simulink model "srmob_lab_model"  (R2018a)
settings: Solver=ode45  StartTime=0.0  StopTime=t_end  FixedStep=t_pp  MaxStep=t_pp  RelTol=1e-3
values from neighbouring files (symbols this model uses):
  inv_J = inv(J)    [srmob_lab_init.m]
  inv_N = inv(N)    [srmob_lab_init.m]
  inv_R_m = inv(R_m)    [srmob_lab_init.m]
  k_c = k_i+50    (= 115.65867657)    [srmob_lab_init.m]
  k_i = (T*omega_0^2) / (K*k_p)    (= 65.6586765699)    [srmob_lab_init.m]
  K_m = [k_m 0; 0 k_m]    [srmob_lab_init.m]
  k_p = (2*T*zeta_0*omega_0 - 1) / K    (= 2.52443181818)    [srmob_lab_init.m]
  q_initial_conditions = [0; 0; -0.5]    [srmob_lab_init.m]
  T_F = 1/k_i    (= 0.0152302795646)    [srmob_lab_init.m]
  u_initial_conditions = [0; 0]    [srmob_lab_init.m]
  u_max = [u_limit; u_limit]    [srmob_lab_init.m]
  u_min = [-u_limit; -u_limit]    [srmob_lab_init.m]
settings Model: Creator=szymon  LastModifiedBy=tomas

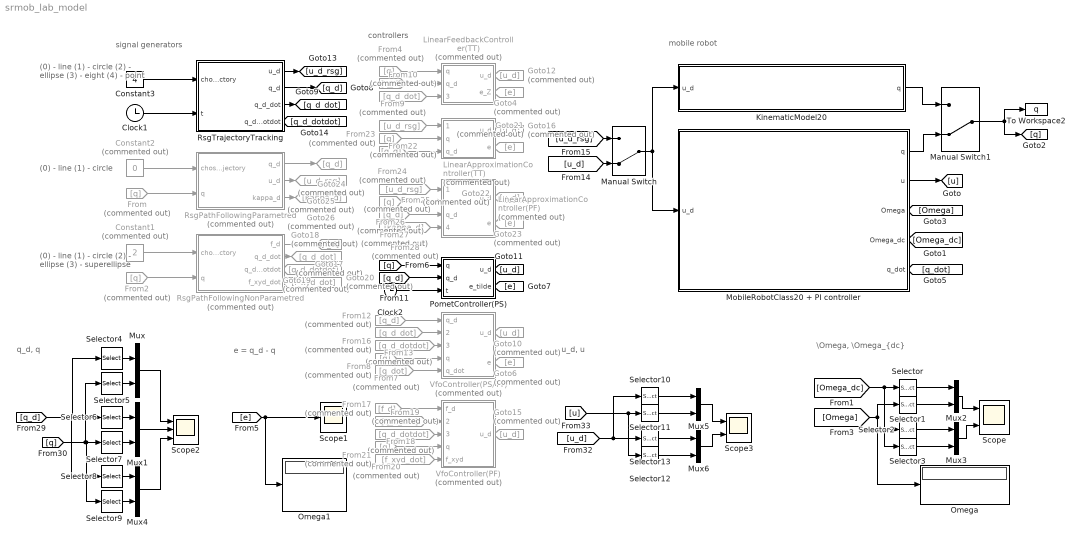
== system srmob_lab_model ==
  note: e = q_d - q
  note: signal generators
  note: controllers
  note: \Omega, \Omega_{dc}
  note: (0) - line
      | (1) - circle
      | (2) - ellipse
      | (3) - eight
      | (4) - point
  note: mobile robot
  note: (0) - line
      | (1) - circle
  note: (0) - line
      | (1) - circle
      | (2) - ellipse
      | (3) - superellipse
  note: q_d, q
  note: u_d, u
  Clock1 : Clock
  Clock2 : Clock
  Constant1 : Constant  Commented=on  Value=2
  Constant2 : Constant  Commented=on  Value=0
  Constant3 : Constant  Value=4
  From{,2,4,7,20,23,26} (7 alike) : From  Commented=on  GotoTag=q
  From10 : From  Commented=on  GotoTag=q_d_dot
  From{9,12,24,27} (4 alike) : From  Commented=on  GotoTag=q_d
  From13 : From  Commented=on  GotoTag=q_d_dot
  From16 : From  Commented=on  GotoTag=q_d_dotdot
  From17 : From  Commented=on  GotoTag=f_d
  From18 : From  Commented=on  GotoTag=q_d_dot
  From19 : From  Commented=on  GotoTag=q_d_dotdot
  From21 : From  Commented=on  GotoTag=f_xyd_dot
  From22 : From  Commented=on  GotoTag=u_d_rsg
  From25 : From  Commented=on  GotoTag=u_d_rsg
  From28 : From  Commented=on  GotoTag=kappa_d
  From8 : From  Commented=on  GotoTag=q_dot
  Goto{10,12,15..16,22} (5 alike) : Goto  Commented=on  GotoTag=u_d
  Goto17 : Goto  Commented=on  GotoTag=f_d
  Goto18 : Goto  Commented=on  GotoTag=q_d_dot
  Goto19 : Goto  Commented=on  GotoTag=q_d_dotdot
  Goto20 : Goto  Commented=on  GotoTag=f_xyd_dot
  Goto{4,6,21,23} (4 alike) : Goto  Commented=on  GotoTag=e
  Goto24 : Goto  Commented=on  GotoTag=q_d
  Goto25 : Goto  Commented=on  GotoTag=u_d_rsg
  Goto26 : Goto  Commented=on  GotoTag=kappa_d
  KinematicModel20 : Subsystem
  LinearApproximationController(PF) : Subsystem  Commented=on
  LinearApproximationController(TT) : Subsystem  Commented=on
  LinearFeedbackController(TT) : Subsystem  Commented=on
  Manual Switch : ManualSwitch  CurrentSetting=0
  Manual Switch1 : ManualSwitch  CurrentSetting=0
  MobileRobotClass20 + PI controller : Subsystem
  Mux{,1..6} (7 alike) : Mux  Inputs=2
  Omega : Display
  Omega1 : Display
  PometController(PS) : Subsystem
  RsgPathFollowingNonParametred : Subsystem  Commented=on
  RsgPathFollowingParametred : Subsystem  Commented=on
  RsgTrajectoryTracking : Subsystem
  Scope : Scope  NumInputPorts=2
  Scope1 : Scope
  Scope2 : Scope  NumInputPorts=3
  Scope3 : Scope  NumInputPorts=2
  Selector{,1,10..11} (4 alike) : Selector  InputPortWidth=2  IndexOptions=Index vector (dialog)  Indices=1  OutputSizes=1
  Selector{2..3,12..13} (4 alike) : Selector  InputPortWidth=2  IndexOptions=Index vector (dialog)  Indices=2  OutputSizes=1
  Selector4 : Selector  InputPortWidth=3  IndexOptions=Index vector (dialog)  Indices=1  OutputSizes=1
  Selector5 : Selector  InputPortWidth=3  IndexOptions=Index vector (dialog)  Indices=1  OutputSizes=1
  Selector6 : Selector  InputPortWidth=3  IndexOptions=Index vector (dialog)  Indices=2  OutputSizes=1
  Selector7 : Selector  InputPortWidth=3  IndexOptions=Index vector (dialog)  Indices=2  OutputSizes=1
  Selector8 : Selector  InputPortWidth=3  IndexOptions=Index vector (dialog)  Indices=3  OutputSizes=1
  Selector9 : Selector  InputPortWidth=3  IndexOptions=Index vector (dialog)  Indices=3  OutputSizes=1
  To Workspace2 : ToWorkspace  VariableName=q  SampleTime=-1
  VfoController(PF) : Subsystem  Commented=on
  VfoController(PS/TT) : Subsystem  Commented=on
  wires:
  Selector/1 -> Mux2/1
  Selector1/1 -> Mux2/2
  Selector2/1 -> Mux3/1
  Selector3/1 -> Mux3/2
  Mux2/1 -> Scope/1
  Clock1/1 -> RsgTrajectoryTracking/2(t)
  From/1 -> RsgPathFollowingParametred/2(q)
  MobileRobotClass20 + PI controller/1(q) -> Manual Switch1/2
  MobileRobotClass20 + PI controller/2(u) -> [u]
  MobileRobotClass20 + PI controller/4(Omega_dc) -> [Omega_dc]
  From2/1 -> RsgPathFollowingNonParametred/2(q)
  MobileRobotClass20 + PI controller/3(Omega) -> [Omega]
  Constant1/1 -> RsgPathFollowingNonParametred/1(chosen_trajectory)
  Constant2/1 -> RsgPathFollowingParametred/1(chosen_trajectory)
  Constant3/1 -> RsgTrajectoryTracking/1(chosen_trajectory)
  Manual Switch1/1 -> To Workspace2/1, [q]
  From4/1 -> LinearFeedbackController(TT)/1(q)
  Manual Switch/1 -> KinematicModel20/1(u_d), MobileRobotClass20 + PI controller/1(u_d)
  LinearFeedbackController(TT)/2(e_Z) -> Goto4/1
  [e] -> Scope1/1, Omega1/1
  Mux3/1 -> Scope/2
  [Omega_dc] -> Selector3/1, Selector/1
  [Omega] -> Omega/1, Selector2/1, Selector1/1
  Clock2/1 -> PometController(PS)/3(t)
  [q] -> PometController(PS)/1(q)
  From7/1 -> VfoController(PS/TT)/4(q)
  PometController(PS)/1(u_d) -> [u_d]
  MobileRobotClass20 + PI controller/5(q_dot) -> [q_dot]
  From8/1 -> VfoController(PS/TT)/5(q_dot)
  VfoController(PS/TT)/2(e) -> Goto6/1
  PometController(PS)/2(e_tilde) -> [e]
  RsgTrajectoryTracking/2(q_d) -> [q_d]
  From9/1 -> LinearFeedbackController(TT)/2(q_d)
  RsgTrajectoryTracking/3(q_d_dot) -> [q_d_dot]
  From10/1 -> LinearFeedbackController(TT)/3(q_d_dot)
  [q_d] -> PometController(PS)/2(q_d)
  From12/1 -> VfoController(PS/TT)/1(q_d)
  From13/1 -> VfoController(PS/TT)/2(q_d_dot)
  VfoController(PS/TT)/1(u_d) -> Goto10/1
  LinearFeedbackController(TT)/1(u_d) -> Goto12/1
  [u_d] -> Manual Switch/2
  RsgTrajectoryTracking/1(u_d) -> [u_d_rsg]
  [u_d_rsg] -> Manual Switch/1
  KinematicModel20/1(q) -> Manual Switch1/1
  RsgTrajectoryTracking/4(q_d_dotdot) -> [q_d_dotdot]
  From16/1 -> VfoController(PS/TT)/3(q_d_dotdot)
  RsgPathFollowingNonParametred/2(q_d_dot) -> Goto18/1
  RsgPathFollowingNonParametred/3(q_d_dotdot) -> Goto19/1
  RsgPathFollowingNonParametred/1(f_d) -> Goto17/1
  From18/1 -> VfoController(PF)/2(q_d_dot)
  From19/1 -> VfoController(PF)/3(q_d_dotdot)
  From17/1 -> VfoController(PF)/1(f_d)
  From20/1 -> VfoController(PF)/4(q)
  RsgPathFollowingNonParametred/4(f_xyd_dot) -> Goto20/1
  From21/1 -> VfoController(PF)/5(f_xyd)
  VfoController(PF)/1(u_d) -> Goto15/1
  From23/1 -> LinearApproximationController(TT)/2(q)
  LinearApproximationController(TT)/1(u_d) -> Goto16/1
  LinearApproximationController(TT)/2(e) -> Goto21/1
  From24/1 -> LinearApproximationController(TT)/3(q_d)
  From22/1 -> LinearApproximationController(TT)/1(u_d_rsg)
  LinearApproximationController(PF)/1(u_d) -> Goto22/1
  LinearApproximationController(PF)/2(e) -> Goto23/1
  RsgPathFollowingParametred/1(q_d) -> Goto24/1
  RsgPathFollowingParametred/2(u_d) -> Goto25/1
  RsgPathFollowingParametred/3(kappa_d) -> Goto26/1
  From25/1 -> LinearApproximationController(PF)/1(u_d_rsg)
  From26/1 -> LinearApproximationController(PF)/2(q)
  From27/1 -> LinearApproximationController(PF)/3(q_d)
  From28/1 -> LinearApproximationController(PF)/4(kappa_d)
  [q_d] -> Selector8/1, Selector4/1, Selector6/1
  Selector4/1 -> Mux/1
  Selector5/1 -> Mux/2
  Mux/1 -> Scope2/1
  Selector7/1 -> Mux1/2
  Mux1/1 -> Scope2/2
  Selector6/1 -> Mux1/1
  Selector9/1 -> Mux4/2
  Mux4/1 -> Scope2/3
  Selector8/1 -> Mux4/1
  [q] -> Selector5/1, Selector9/1, Selector7/1
  Selector13/1 -> Mux6/1
  Selector10/1 -> Mux5/1
  Mux6/1 -> Scope3/2
  Selector11/1 -> Mux5/2
  Mux5/1 -> Scope3/1
  Selector12/1 -> Mux6/2
  [u_d] -> Selector10/1, Selector13/1
  [u] -> Selector12/1, Selector11/1

== system srmob_lab_model/KinematicModel20 ==
  u_d : Inport
  Demux : Demux  Outputs=3
  Integrator : Integrator  InitialCondition=q_initial_conditions
  KinematicModel : MATLABFcn  MATLABFcn=KinematicModel
  Mux : Mux  Inputs=2
  Mux1 : Mux  Inputs=3
  q : Outport
  wires:
  KinematicModel/1 -> Integrator/1  "q'"
  Mux/1 -> KinematicModel/1
  u_d/1 -> Mux/2
  Integrator/1 -> Demux/1  "q"
  Demux/1 -> Mux/1, Mux1/1  "theta"
  Demux/3 -> Mux1/3  "y"
  Demux/2 -> Mux1/2  "x"
  Mux1/1 -> q/1

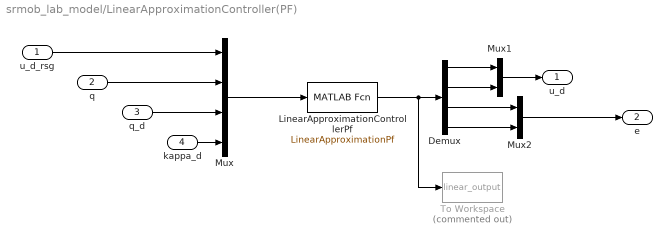
== system srmob_lab_model/LinearApproximationController(PF) ==
  u_d_rsg : Inport
  q : Inport  Port=2
  q_d : Inport  Port=3
  kappa_d : Inport  Port=4
  Demux : Demux
  LinearApproximationControllerPf : MATLABFcn  MATLABFcn=LinearApproximationPf
  Mux : Mux
  Mux1 : Mux  Inputs=2
  Mux2 : Mux  Inputs=2
  To Workspace : ToWorkspace  Commented=on  VariableName=linear_output  SampleTime=-1
  u_d : Outport
  e : Outport  Port=2
  wires:
  Mux/1 -> LinearApproximationControllerPf/1
  q_d/1 -> Mux/3
  LinearApproximationControllerPf/1 -> Demux/1, To Workspace/1
  Demux/1 -> Mux1/1
  Demux/2 -> Mux1/2
  Mux2/1 -> e/1
  Mux1/1 -> u_d/1
  u_d_rsg/1 -> Mux/1
  q/1 -> Mux/2
  kappa_d/1 -> Mux/4
  Demux/4 -> Mux2/2
  Demux/3 -> Mux2/1

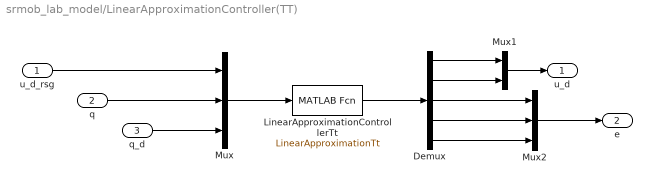
== system srmob_lab_model/LinearApproximationController(TT) ==
  u_d_rsg : Inport
  q : Inport  Port=2
  q_d : Inport  Port=3
  Demux : Demux  Outputs=5
  LinearApproximationControllerTt : MATLABFcn  MATLABFcn=LinearApproximationTt
  Mux : Mux  Inputs=3
  Mux1 : Mux  Inputs=2
  Mux2 : Mux  Inputs=3
  u_d : Outport
  e : Outport  Port=2
  wires:
  Mux/1 -> LinearApproximationControllerTt/1
  q_d/1 -> Mux/3
  LinearApproximationControllerTt/1 -> Demux/1
  Demux/1 -> Mux1/1
  Demux/2 -> Mux1/2
  Demux/3 -> Mux2/1
  Demux/4 -> Mux2/2
  Mux2/1 -> e/1
  Mux1/1 -> u_d/1
  u_d_rsg/1 -> Mux/1
  q/1 -> Mux/2
  Demux/5 -> Mux2/3

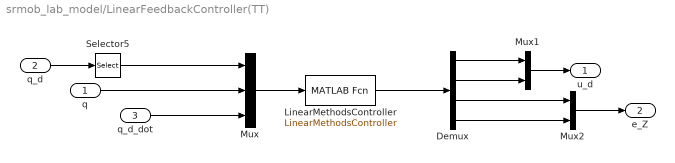
== system srmob_lab_model/LinearFeedbackController(TT) ==
  q : Inport
  q_d : Inport  Port=2
  q_d_dot : Inport  Port=3
  Demux : Demux
  LinearMethodsController : MATLABFcn  MATLABFcn=LinearMethodsController
  Mux : Mux  Inputs=3
  Mux1 : Mux  Inputs=2
  Mux2 : Mux  Inputs=2
  Selector5 : Selector  InputPortWidth=3  IndexOptions=Index vector (dialog)  Indices=[2 3]  OutputSizes=1
  u_d : Outport
  e_Z : Outport  Port=2
  wires:
  Mux/1 -> LinearMethodsController/1
  q/1 -> Mux/2
  q_d/1 -> Selector5/1
  LinearMethodsController/1 -> Demux/1
  q_d_dot/1 -> Mux/3
  Demux/1 -> Mux1/1
  Demux/2 -> Mux1/2
  Demux/3 -> Mux2/1
  Demux/4 -> Mux2/2
  Mux2/1 -> e_Z/1
  Mux1/1 -> u_d/1
  Selector5/1 -> Mux/1

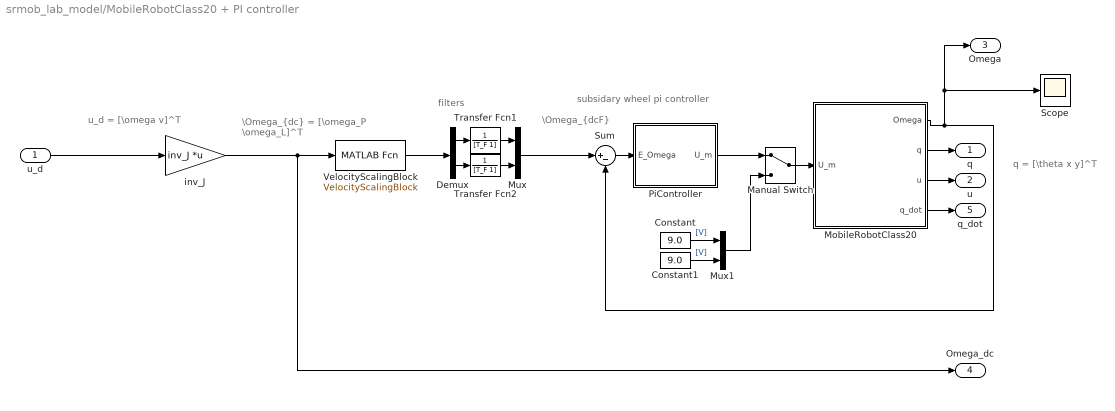
== system srmob_lab_model/MobileRobotClass20 + PI controller ==
  note: q = [\theta x y]^T
  note: u_d = [\omega v]^T
  note: \Omega_{dc} = [\omega_P \omega_L]^T
  note: \Omega_{dcF}
  note: subsidary wheel pi controller
  note: filters
  u_d : Inport
  Constant : Constant  Value=9.0
  Constant1 : Constant  Value=9.0
  Demux : Demux  Outputs=2
  Manual Switch : ManualSwitch
  MobileRobotClass20 : Subsystem
  Mux : Mux  Inputs=2
  Mux1 : Mux  Inputs=2
  PiController : Subsystem
  Scope : Scope
  Sum : Sum  Inputs=|+-
  Transfer Fcn1 : TransferFcn  Numerator=1  Denominator=[T_F 1]
  Transfer Fcn2 : TransferFcn  Numerator=1  Denominator=[T_F 1]
  VelocityScalingBlock : MATLABFcn  MATLABFcn=VelocityScalingBlock
  inv_J : Gain  Gain=inv_J  Multiplication=Matrix(K*u)
  q : Outport
  u : Outport  Port=2
  Omega : Outport  Port=3
  Omega_dc : Outport  Port=4
  q_dot : Outport  Port=5
  wires:
  Demux/1 -> Transfer Fcn1/1
  Transfer Fcn1/1 -> Mux/1
  Transfer Fcn2/1 -> Mux/2
  u_d/1 -> inv_J/1
  Constant/1 -> Mux1/1  "[V]"
  MobileRobotClass20/2(q) -> q/1
  Demux/2 -> Transfer Fcn2/1
  Manual Switch/1 -> MobileRobotClass20/1(U_m)
  Sum/1 -> PiController/1(E_Omega)
  MobileRobotClass20/3(u) -> u/1
  MobileRobotClass20/1(Omega) -> Omega/1, Scope/1, Sum/2
  Mux1/1 -> Manual Switch/2
  PiController/1(U_m) -> Manual Switch/1
  Mux/1 -> Sum/1
  VelocityScalingBlock/1 -> Demux/1
  Constant1/1 -> Mux1/2  "[V]"
  inv_J/1 -> Omega_dc/1, VelocityScalingBlock/1
  MobileRobotClass20/4(q_dot) -> q_dot/1

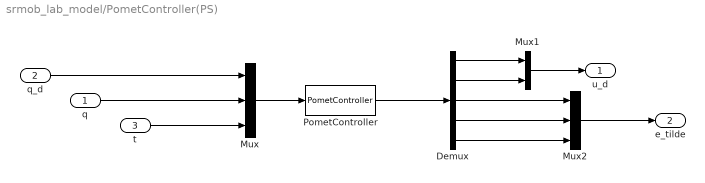
== system srmob_lab_model/PometController(PS) ==
  q : Inport
  q_d : Inport  Port=2
  t : Inport  Port=3
  Demux : Demux  Outputs=5
  Mux : Mux  Inputs=3
  Mux1 : Mux  Inputs=2
  Mux2 : Mux  Inputs=3
  PometController : MATLABFcn  MATLABFcn=PometController
  u_d : Outport
  e_tilde : Outport  Port=2
  wires:
  Mux/1 -> PometController/1
  q/1 -> Mux/2
  q_d/1 -> Mux/1
  PometController/1 -> Demux/1
  t/1 -> Mux/3
  Demux/1 -> Mux1/1
  Demux/2 -> Mux1/2
  Demux/3 -> Mux2/1
  Demux/4 -> Mux2/2
  Mux2/1 -> e_tilde/1
  Mux1/1 -> u_d/1
  Demux/5 -> Mux2/3

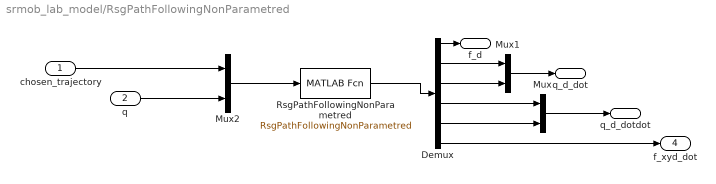
== system srmob_lab_model/RsgPathFollowingNonParametred ==
  chosen_trajectory : Inport
  q : Inport  Port=2
  Demux : Demux  Outputs=6
  Mux : Mux  Inputs=2
  Mux1 : Mux  Inputs=2
  Mux2 : Mux  Inputs=2
  RsgPathFollowingNonParametred : MATLABFcn  MATLABFcn=RsgPathFollowingNonParametred
  f_d : Outport
  q_d_dot : Outport  Port=2
  q_d_dotdot : Outport  Port=3
  f_xyd_dot : Outport  Port=4
  wires:
  RsgPathFollowingNonParametred/1 -> Demux/1
  q/1 -> Mux2/2
  chosen_trajectory/1 -> Mux2/1
  Mux2/1 -> RsgPathFollowingNonParametred/1
  Mux/1 -> q_d_dotdot/1
  Demux/2 -> Mux1/1
  Demux/3 -> Mux1/2
  Demux/4 -> Mux/1
  Demux/5 -> Mux/2
  Demux/1 -> f_d/1
  Mux1/1 -> q_d_dot/1
  Demux/6 -> f_xyd_dot/1

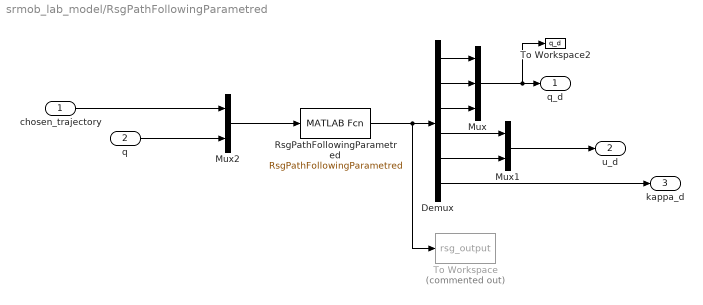
== system srmob_lab_model/RsgPathFollowingParametred ==
  chosen_trajectory : Inport
  q : Inport  Port=2
  Demux : Demux  Outputs=6
  Mux : Mux  Inputs=3
  Mux1 : Mux  Inputs=2
  Mux2 : Mux  Inputs=2
  RsgPathFollowingParametred : MATLABFcn  MATLABFcn=RsgPathFollowingParametred
  To Workspace : ToWorkspace  Commented=on  VariableName=rsg_output  SampleTime=-1
  To Workspace2 : ToWorkspace  VariableName=q_d  SampleTime=-1
  q_d : Outport
  u_d : Outport  Port=2
  kappa_d : Outport  Port=3
  wires:
  RsgPathFollowingParametred/1 -> Demux/1, To Workspace/1
  Demux/1 -> Mux/1
  Demux/2 -> Mux/2
  Demux/3 -> Mux/3
  Demux/5 -> Mux1/2
  Demux/4 -> Mux1/1
  Mux1/1 -> u_d/1
  q/1 -> Mux2/2
  chosen_trajectory/1 -> Mux2/1
  Mux2/1 -> RsgPathFollowingParametred/1
  Demux/6 -> kappa_d/1
  Mux/1 -> To Workspace2/1, q_d/1

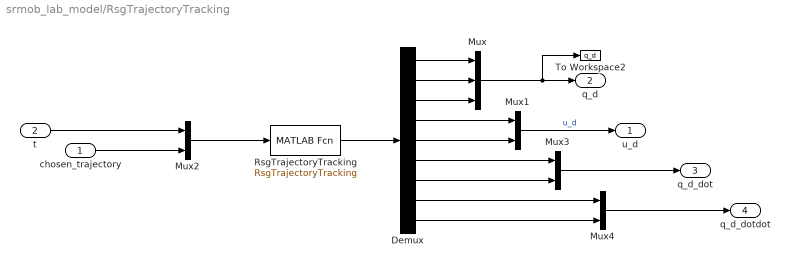
== system srmob_lab_model/RsgTrajectoryTracking ==
  chosen_trajectory : Inport
  t : Inport  Port=2
  Demux : Demux  Outputs=9
  Mux : Mux  Inputs=3
  Mux{1..4} (4 alike) : Mux  Inputs=2
  RsgTrajectoryTracking : MATLABFcn  MATLABFcn=RsgTrajectoryTracking
  To Workspace2 : ToWorkspace  VariableName=q_d  SampleTime=-1
  u_d : Outport
  q_d : Outport  Port=2
  q_d_dot : Outport  Port=3
  q_d_dotdot : Outport  Port=4
  wires:
  t/1 -> Mux2/1
  RsgTrajectoryTracking/1 -> Demux/1
  Demux/1 -> Mux/1
  Demux/2 -> Mux/2
  Demux/3 -> Mux/3
  Mux/1 -> To Workspace2/1, q_d/1
  Demux/5 -> Mux1/2
  Demux/4 -> Mux1/1
  Mux1/1 -> u_d/1  "u_d"
  Mux2/1 -> RsgTrajectoryTracking/1
  chosen_trajectory/1 -> Mux2/2
  Demux/7 -> Mux3/2
  Demux/6 -> Mux3/1
  Mux3/1 -> q_d_dot/1
  Demux/9 -> Mux4/2
  Demux/8 -> Mux4/1
  Mux4/1 -> q_d_dotdot/1

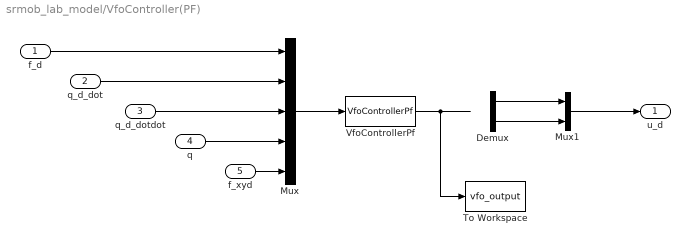
== system srmob_lab_model/VfoController(PF) ==
  f_d : Inport
  q_d_dot : Inport  Port=2
  q_d_dotdot : Inport  Port=3
  q : Inport  Port=4
  f_xyd : Inport  Port=5
  Demux : Demux  Outputs=2
  Mux : Mux  Inputs=5
  Mux1 : Mux  Inputs=2
  To Workspace : ToWorkspace  VariableName=vfo_output  SampleTime=-1
  VfoControllerPf : MATLABFcn  MATLABFcn=VfoControllerPf
  u_d : Outport
  wires:
  Mux/1 -> VfoControllerPf/1
  q_d_dot/1 -> Mux/2
  f_d/1 -> Mux/1
  VfoControllerPf/1 -> To Workspace/1
  q_d_dotdot/1 -> Mux/3
  Demux/1 -> Mux1/1
  Demux/2 -> Mux1/2
  Mux1/1 -> u_d/1
  q/1 -> Mux/4
  f_xyd/1 -> Mux/5

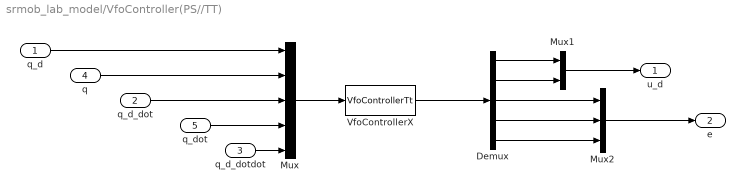
== system srmob_lab_model/VfoController(PS//TT) ==
  q_d : Inport
  q_d_dot : Inport  Port=2
  q_d_dotdot : Inport  Port=3
  q : Inport  Port=4
  q_dot : Inport  Port=5
  Demux : Demux  Outputs=5
  Mux : Mux  Inputs=5
  Mux1 : Mux  Inputs=2
  Mux2 : Mux  Inputs=3
  VfoControllerX : MATLABFcn  MATLABFcn=VfoControllerTt
  u_d : Outport
  e : Outport  Port=2
  wires:
  Mux/1 -> VfoControllerX/1
  q/1 -> Mux/2
  q_d/1 -> Mux/1
  VfoControllerX/1 -> Demux/1
  q_d_dot/1 -> Mux/3
  Demux/1 -> Mux1/1
  Demux/2 -> Mux1/2
  q_dot/1 -> Mux/4
  Mux1/1 -> u_d/1
  Demux/4 -> Mux2/2
  Demux/3 -> Mux2/1
  Mux2/1 -> e/1
  q_d_dotdot/1 -> Mux/5
  Demux/5 -> Mux2/3

== system srmob_lab_model/MobileRobotClass20 + PI controller/MobileRobotClass20 ==
  U_m : Inport
  DynamicModel : Subsystem
  KinematicModel : Subsystem
  Omega : Outport
  q : Outport  Port=2
  u : Outport  Port=3
  q_dot : Outport  Port=4
  wires:
  KinematicModel/1(q) -> q/1
  DynamicModel/1(Omega) -> Omega/1
  U_m/1 -> DynamicModel/1(U_m)
  DynamicModel/2(u_d) -> u/1, KinematicModel/1(u_d)
  KinematicModel/2(q_dot) -> q_dot/1

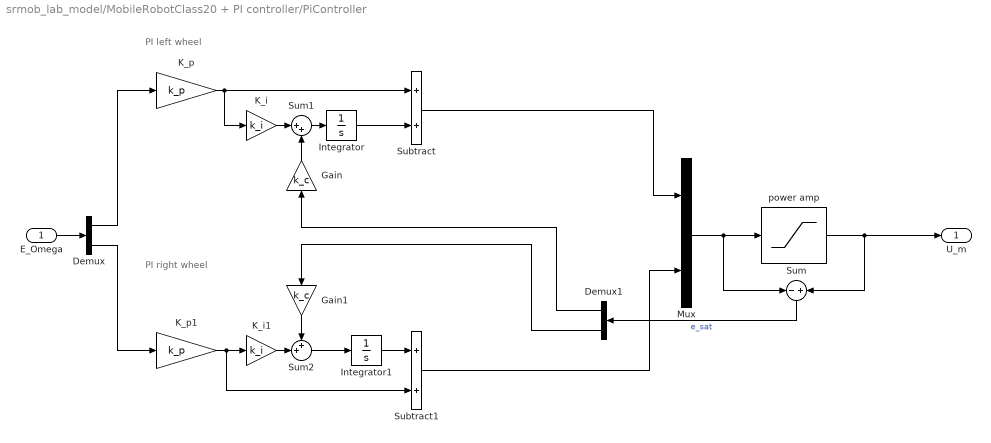
== system srmob_lab_model/MobileRobotClass20 + PI controller/PiController ==
  note: PI left wheel
  note: PI right wheel
  E_Omega : Inport
  Demux : Demux  Outputs=2
  Demux1 : Demux  Outputs=2
  Gain : Gain  Gain=k_c
  Gain1 : Gain  Gain=k_c
  Integrator : Integrator  InitialCondition=[0]
  Integrator1 : Integrator  InitialCondition=[0]
  K_i : Gain  Gain=k_i
  K_i1 : Gain  Gain=k_i
  K_p : Gain  Gain=k_p
  K_p1 : Gain  Gain=k_p
  Mux : Mux  Inputs=2
  Subtract : Sum
  Subtract1 : Sum
  Sum : Sum  Inputs=-+
  Sum1 : Sum  Inputs=|++
  Sum2 : Sum  Inputs=++|
  power amp : Saturate  UpperLimit=u_max  LowerLimit=u_min
  U_m : Outport
  wires:
  Demux/1 -> K_p/1
  Subtract/1 -> Mux/1
  K_i/1 -> Sum1/1
  K_p/1 -> K_i/1, Subtract/1
  Integrator/1 -> Subtract/2
  Demux/2 -> K_p1/1
  Subtract1/1 -> Mux/2
  K_p1/1 -> Subtract1/2, K_i1/1
  Integrator1/1 -> Subtract1/1
  Mux/1 -> Sum/1, power amp/1
  E_Omega/1 -> Demux/1
  power amp/1 -> Sum/2, U_m/1
  Sum/1 -> Demux1/1  "e_sat"
  Sum1/1 -> Integrator/1
  Demux1/1 -> Gain/1
  Sum2/1 -> Integrator1/1
  Gain/1 -> Sum1/2
  Demux1/2 -> Gain1/1
  K_i1/1 -> Sum2/2
  Gain1/1 -> Sum2/1

== system srmob_lab_model/MobileRobotClass20 + PI controller/MobileRobotClass20/DynamicModel ==
  U_m : Inport
  DynamicModel : MATLABFcn  MATLABFcn=DynamicModel
  Integrator : Integrator  InitialCondition=u_initial_conditions
  Mux : Mux  Inputs=2
  VoltageTorqueCalc : Subsystem
  inv_J : Gain  Gain=inv_J  Multiplication=Matrix(K*u) (u vector)
  power amp : Saturate  UpperLimit=u_max  LowerLimit=u_min
  Omega : Outport
  u_d : Outport  Port=2
  wires:
  Mux/1 -> DynamicModel/1
  DynamicModel/1 -> Integrator/1  "u'_d"
  Integrator/1 -> Mux/1, VoltageTorqueCalc/1(u), inv_J/1, u_d/1  "u"
  U_m/1 -> power amp/1
  inv_J/1 -> Omega/1
  VoltageTorqueCalc/1(T_m) -> Mux/2
  power amp/1 -> VoltageTorqueCalc/2(U_m)

== system srmob_lab_model/MobileRobotClass20 + PI controller/MobileRobotClass20/KinematicModel ==
  u_d : Inport
  Demux : Demux  Outputs=3
  Integrator : Integrator  InitialCondition=q_initial_conditions
  KinematicModel : MATLABFcn  MATLABFcn=KinematicModel
  Mux : Mux  Inputs=2
  Mux1 : Mux  Inputs=3
  q : Outport
  q_dot : Outport  Port=2
  wires:
  KinematicModel/1 -> q_dot/1, Integrator/1  "q'"
  Mux/1 -> KinematicModel/1
  u_d/1 -> Mux/2
  Integrator/1 -> Demux/1  "q"
  Demux/1 -> Mux/1, Mux1/1  "theta"
  Demux/3 -> Mux1/3  "y"
  Demux/2 -> Mux1/2  "x"
  Mux1/1 -> q/1

== system srmob_lab_model/MobileRobotClass20 + PI controller/MobileRobotClass20/DynamicModel/VoltageTorqueCalc ==
  u : Inport
  U_m : Inport  Port=2
  Gain : Gain  Gain=inv_N  Multiplication=Matrix(K*u) (u vector)
  Gain1 : Gain  Gain=K_m  Multiplication=Matrix(K*u) (u vector)
  K_m : Gain  Gain=K_m  Multiplication=Matrix(K*u) (u vector)
  Sum : Sum  Inputs=|+-
  inv_J : Gain  Gain=inv_J  Multiplication=Matrix(K*u) (u vector)
  inv_R : Gain  Gain=inv_R_m  Multiplication=Matrix(K*u) (u vector)
  T_m : Outport
  wires:
  inv_R/1 -> K_m/1  "i_m"
  Gain/1 -> Gain1/1  "Omega_m"
  inv_J/1 -> Gain/1  "Omega"
  Sum/1 -> inv_R/1
  Gain1/1 -> Sum/2  "E_m"
  K_m/1 -> T_m/1
  u/1 -> inv_J/1
  U_m/1 -> Sum/1
